simulink library "DatalogHandler"  (R2016b)
settings: Solver=VariableStepAuto  StartTime=0.0  StopTime=10.0  RelTol=1e-3
libraries: VariousLibrary x6, ConversionsLibrary x6, slrtlib x1
(part 2 of 2)

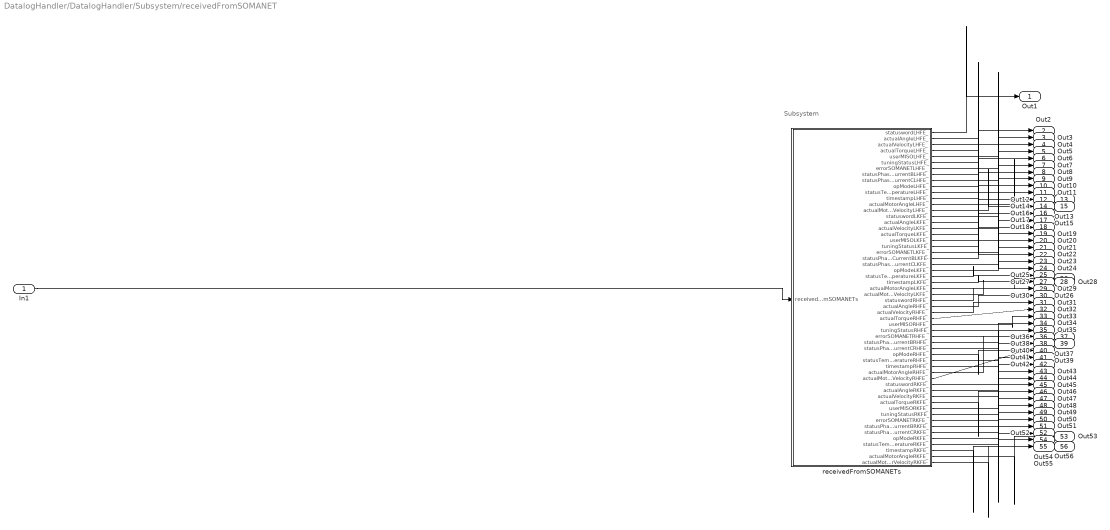
== system DatalogHandler/DatalogHandler/Subsystem/receivedFromSOMANET ==
  note: Subsystem
  In1 : Inport
  receivedFromSOMANETs : Subsystem
  Out1 : Outport
  Out2 : Outport  Port=2
  Out3 : Outport  Port=3
  Out4 : Outport  Port=4
  Out5 : Outport  Port=5
  Out6 : Outport  Port=6
  Out7 : Outport  Port=7
  Out8 : Outport  Port=8
  Out9 : Outport  Port=9
  Out10 : Outport  Port=10
  Out11 : Outport  Port=11
  Out12 : Outport  Port=12
  Out13 : Outport  Port=13
  Out14 : Outport  Port=14
  Out15 : Outport  Port=15
  Out16 : Outport  Port=16
  Out17 : Outport  Port=17
  Out18 : Outport  Port=18
  Out19 : Outport  Port=19
  Out20 : Outport  Port=20
  Out21 : Outport  Port=21
  Out22 : Outport  Port=22
  Out23 : Outport  Port=23
  Out24 : Outport  Port=24
  Out25 : Outport  Port=25
  Out26 : Outport  Port=26
  Out27 : Outport  Port=27
  Out28 : Outport  Port=28
  Out29 : Outport  Port=29
  Out30 : Outport  Port=30
  Out31 : Outport  Port=31
  Out32 : Outport  Port=32
  Out33 : Outport  Port=33
  Out34 : Outport  Port=34
  Out35 : Outport  Port=35
  Out36 : Outport  Port=36
  Out37 : Outport  Port=37
  Out38 : Outport  Port=38
  Out39 : Outport  Port=39
  Out40 : Outport  Port=40
  Out41 : Outport  Port=41
  Out42 : Outport  Port=42
  Out43 : Outport  Port=43
  Out44 : Outport  Port=44
  Out45 : Outport  Port=45
  Out46 : Outport  Port=46
  Out47 : Outport  Port=47
  Out48 : Outport  Port=48
  Out49 : Outport  Port=49
  Out50 : Outport  Port=50
  Out51 : Outport  Port=51
  Out52 : Outport  Port=52
  Out53 : Outport  Port=53
  Out54 : Outport  Port=54
  Out55 : Outport  Port=55
  Out56 : Outport  Port=56
  wires:
  receivedFromSOMANETs/34(tuningStatusRHFE_) -> Out34/1
  receivedFromSOMANETs/49(errorSOMANETRKFE_) -> Out49/1
  receivedFromSOMANETs/53(statusTemperatureRKFE_) -> Out54/1
  receivedFromSOMANETs/48(tuningStatusRKFE_) -> Out48/1
  receivedFromSOMANETs/38(opModeRHFE_) -> Out40/1
  receivedFromSOMANETs/51(statusPhaseCurrentCRKFE_) -> Out51/1
  receivedFromSOMANETs/39(statusTemperatureRHFE_) -> Out41/1
  receivedFromSOMANETs/47(userMISORKFE_) -> Out47/1
  receivedFromSOMANETs/45(actualVelocityRKFE_) -> Out45/1
  receivedFromSOMANETs/32(actualTorqueRHFE_) -> Out32/1
  receivedFromSOMANETs/46(actualTorqueRKFE_) -> Out46/1
  receivedFromSOMANETs/31(actualVelocityRHFE_) -> Out31/1
  receivedFromSOMANETs/44(actualAngleRKFE_) -> Out44/1
  receivedFromSOMANETs/43(statuswordRKFE_) -> Out43/1
  receivedFromSOMANETs/33(userMISORHFE_) -> Out33/1
  receivedFromSOMANETs/35(errorSOMANETRHFE_) -> Out35/1
  receivedFromSOMANETs/54(timestampRKFE_) -> Out55/1
  receivedFromSOMANETs/50(statusPhaseCurrentBRKFE_) -> Out50/1
  receivedFromSOMANETs/37(statusPhaseCurrentCRHFE_) -> Out38/1
  receivedFromSOMANETs/40(timestampRHFE_) -> Out42/1
  receivedFromSOMANETs/52(opModeRKFE_) -> Out52/1
  receivedFromSOMANETs/36(statusPhaseCurrentBRHFE_) -> Out36/1
  receivedFromSOMANETs/30(actualAngleRHFE_) -> Out30/1
  receivedFromSOMANETs/18(actualTorqueLKFE_) -> Out18/1
  receivedFromSOMANETs/1(statuswordLHFE_) -> Out1/1
  receivedFromSOMANETs/2(actualAngleLHFE_) -> Out2/1
  receivedFromSOMANETs/17(actualVelocityLKFE_) -> Out17/1
  receivedFromSOMANETs/11(statusTemperatureLHFE_) -> Out11/1
  receivedFromSOMANETs/10(opModeLHFE_) -> Out10/1
  receivedFromSOMANETs/21(errorSOMANETLKFE_) -> Out21/1
  receivedFromSOMANETs/15(statuswordLKFE_) -> Out14/1
  receivedFromSOMANETs/8(statusPhaseCurrentBLHFE_) -> Out8/1
  receivedFromSOMANETs/4(actualTorqueLHFE_) -> Out4/1
  receivedFromSOMANETs/12(timestampLHFE_) -> Out12/1
  receivedFromSOMANETs/5(userMISOLHFE_) -> Out5/1
  receivedFromSOMANETs/29(statuswordRHFE_) -> Out29/1
  receivedFromSOMANETs/24(opModeLKFE_) -> Out24/1
  receivedFromSOMANETs/3(actualVelocityLHFE_) -> Out3/1
  receivedFromSOMANETs/7(errorSOMANETLHFE_) -> Out7/1
  receivedFromSOMANETs/20(tuningStatusLKFE_) -> Out20/1
  receivedFromSOMANETs/9(statusPhaseCurrentCLHFE_) -> Out9/1
  receivedFromSOMANETs/26(timestampLKFE_) -> Out27/1
  receivedFromSOMANETs/6(tuningStatusLHFE_) -> Out6/1
  receivedFromSOMANETs/25(statusTemperatureLKFE_) -> Out25/1
  receivedFromSOMANETs/23(statusPhaseCurrentCLKFE_) -> Out23/1
  receivedFromSOMANETs/22(statusPhaseCurrentBLKFE-) -> Out22/1
  receivedFromSOMANETs/19(userMISOLKFE_) -> Out19/1
  receivedFromSOMANETs/16(actualAngleLKFE_) -> Out16/1
  receivedFromSOMANETs/13(actualMotorAngleLHFE_) -> Out13/1
  receivedFromSOMANETs/14(actualMotorVelocityLHFE_) -> Out15/1
  receivedFromSOMANETs/56(actualMotorVelocityRKFE-) -> Out56/1
  receivedFromSOMANETs/27(actualMotorAngleLKFE_) -> Out26/1
  receivedFromSOMANETs/55(actualMotorAngleRKFE_) -> Out53/1
  receivedFromSOMANETs/28(actualMotorVelocityLKFE_) -> Out28/1
  receivedFromSOMANETs/42(actualMotorVelocityRHFE_) -> Out39/1
  receivedFromSOMANETs/41(actualMotorAngleRHFE_) -> Out37/1
  In1/1 -> receivedFromSOMANETs/1(receivedFromSOMANETs)

== system DatalogHandler/DatalogHandler/Subsystem/sendToInputDevice ==
  In1 : Inport
  Bus Selector7 : BusSelector  OutputSignals=state,message
  messageToInputDevice : DataTypeConversion  OutDataTypeStr=double  RndMeth=Nearest
  stateToInputDevice : DataTypeConversion  OutDataTypeStr=double  RndMeth=Nearest
  Out1 : Outport
  Out2 : Outport  Port=2
  wires:
  messageToInputDevice/1 -> Out2/1
  stateToInputDevice/1 -> Out1/1
  In1/1 -> Bus Selector7/1
  Bus Selector7/1 -> stateToInputDevice/1  "<state>"
  Bus Selector7/2 -> messageToInputDevice/1  "<message>"

== system DatalogHandler/DatalogHandler/Subsystem/sendToPowerElectronics ==
  In1 : Inport
  Bus Selector9 : BusSelector  OutputSignals=sendToPDB.masterOP
  masterOP : DataTypeConversion  OutDataTypeStr=double  RndMeth=Nearest
  Out1 : Outport
  wires:
  masterOP/1 -> Out1/1
  In1/1 -> Bus Selector9/1
  Bus Selector9/1 -> masterOP/1  "<masterOP>"

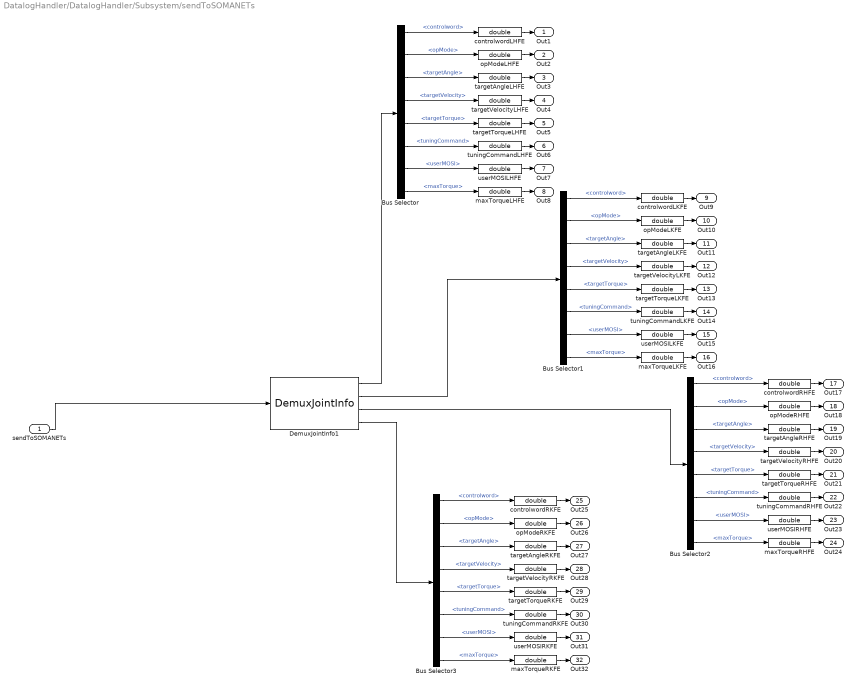
== system DatalogHandler/DatalogHandler/Subsystem/sendToSOMANETs ==
  sendToSOMANETs : Inport
  Bus Selector{,1..3} (4 alike) : BusSelector  OutputSignals=controlword,opMode,targetAngle,targetVelocity,targetTorque,tuningCommand,userMOSI,maxTorque
  DemuxJointInfo1 : VariousLibrary/DemuxJointInfo
  controlwordLHFE : DataTypeConversion  OutDataTypeStr=double  RndMeth=Nearest
  controlwordLKFE : DataTypeConversion  OutDataTypeStr=double  RndMeth=Nearest
  controlwordRHFE : DataTypeConversion  OutDataTypeStr=double  RndMeth=Nearest
  controlwordRKFE : DataTypeConversion  OutDataTypeStr=double  RndMeth=Nearest
  maxTorqueLHFE : DataTypeConversion  OutDataTypeStr=double  RndMeth=Nearest
  maxTorqueLKFE : DataTypeConversion  OutDataTypeStr=double  RndMeth=Nearest
  maxTorqueRHFE : DataTypeConversion  OutDataTypeStr=double  RndMeth=Nearest
  maxTorqueRKFE : DataTypeConversion  OutDataTypeStr=double  RndMeth=Nearest
  opModeLHFE : DataTypeConversion  OutDataTypeStr=double  RndMeth=Nearest
  opModeLKFE : DataTypeConversion  OutDataTypeStr=double  RndMeth=Nearest
  opModeRHFE : DataTypeConversion  OutDataTypeStr=double  RndMeth=Nearest
  opModeRKFE : DataTypeConversion  OutDataTypeStr=double  RndMeth=Nearest
  targetAngleLHFE : DataTypeConversion  OutDataTypeStr=double  RndMeth=Nearest
  targetAngleLKFE : DataTypeConversion  OutDataTypeStr=double  RndMeth=Nearest
  targetAngleRHFE : DataTypeConversion  OutDataTypeStr=double  RndMeth=Nearest
  targetAngleRKFE : DataTypeConversion  OutDataTypeStr=double  RndMeth=Nearest
  targetTorqueLHFE : DataTypeConversion  OutDataTypeStr=double  RndMeth=Nearest
  targetTorqueLKFE : DataTypeConversion  OutDataTypeStr=double  RndMeth=Nearest
  targetTorqueRHFE : DataTypeConversion  OutDataTypeStr=double  RndMeth=Nearest
  targetTorqueRKFE : DataTypeConversion  OutDataTypeStr=double  RndMeth=Nearest
  targetVelocityLHFE : DataTypeConversion  OutDataTypeStr=double  RndMeth=Nearest
  targetVelocityLKFE : DataTypeConversion  OutDataTypeStr=double  RndMeth=Nearest
  targetVelocityRHFE : DataTypeConversion  OutDataTypeStr=double  RndMeth=Nearest
  targetVelocityRKFE : DataTypeConversion  OutDataTypeStr=double  RndMeth=Nearest
  tuningCommandLHFE : DataTypeConversion  OutDataTypeStr=double  RndMeth=Nearest
  tuningCommandLKFE : DataTypeConversion  OutDataTypeStr=double  RndMeth=Nearest
  tuningCommandRHFE : DataTypeConversion  OutDataTypeStr=double  RndMeth=Nearest
  tuningCommandRKFE : DataTypeConversion  OutDataTypeStr=double  RndMeth=Nearest
  userMOSILHFE : DataTypeConversion  OutDataTypeStr=double  RndMeth=Nearest
  userMOSILKFE : DataTypeConversion  OutDataTypeStr=double  RndMeth=Nearest
  userMOSIRHFE : DataTypeConversion  OutDataTypeStr=double  RndMeth=Nearest
  userMOSIRKFE : DataTypeConversion  OutDataTypeStr=double  RndMeth=Nearest
  Out1 : Outport
  Out2 : Outport  Port=2
  Out3 : Outport  Port=3
  Out4 : Outport  Port=4
  Out5 : Outport  Port=5
  Out6 : Outport  Port=6
  Out7 : Outport  Port=7
  Out8 : Outport  Port=8
  Out9 : Outport  Port=9
  Out10 : Outport  Port=10
  Out11 : Outport  Port=11
  Out12 : Outport  Port=12
  Out13 : Outport  Port=13
  Out14 : Outport  Port=14
  Out15 : Outport  Port=15
  Out16 : Outport  Port=16
  Out17 : Outport  Port=17
  Out18 : Outport  Port=18
  Out19 : Outport  Port=19
  Out20 : Outport  Port=20
  Out21 : Outport  Port=21
  Out22 : Outport  Port=22
  Out23 : Outport  Port=23
  Out24 : Outport  Port=24
  Out25 : Outport  Port=25
  Out26 : Outport  Port=26
  Out27 : Outport  Port=27
  Out28 : Outport  Port=28
  Out29 : Outport  Port=29
  Out30 : Outport  Port=30
  Out31 : Outport  Port=31
  Out32 : Outport  Port=32
  wires:
  DemuxJointInfo1/4 -> Bus Selector3/1
  maxTorqueRKFE/1 -> Out32/1
  userMOSIRKFE/1 -> Out31/1
  tuningCommandRKFE/1 -> Out30/1
  targetTorqueRKFE/1 -> Out29/1
  targetVelocityRKFE/1 -> Out28/1
  targetAngleRKFE/1 -> Out27/1
  opModeRKFE/1 -> Out26/1
  controlwordRKFE/1 -> Out25/1
  Bus Selector3/8 -> maxTorqueRKFE/1  "<maxTorque>"
  Bus Selector3/7 -> userMOSIRKFE/1  "<userMOSI>"
  Bus Selector3/6 -> tuningCommandRKFE/1  "<tuningCommand>"
  Bus Selector3/5 -> targetTorqueRKFE/1  "<targetTorque>"
  Bus Selector3/4 -> targetVelocityRKFE/1  "<targetVelocity>"
  Bus Selector3/3 -> targetAngleRKFE/1  "<targetAngle>"
  Bus Selector3/2 -> opModeRKFE/1  "<opMode>"
  Bus Selector3/1 -> controlwordRKFE/1  "<controlword>"
  maxTorqueRHFE/1 -> Out24/1
  userMOSIRHFE/1 -> Out23/1
  tuningCommandRHFE/1 -> Out22/1
  targetTorqueRHFE/1 -> Out21/1
  targetVelocityRHFE/1 -> Out20/1
  targetAngleRHFE/1 -> Out19/1
  opModeRHFE/1 -> Out18/1
  controlwordRHFE/1 -> Out17/1
  Bus Selector2/8 -> maxTorqueRHFE/1  "<maxTorque>"
  Bus Selector2/7 -> userMOSIRHFE/1  "<userMOSI>"
  Bus Selector2/6 -> tuningCommandRHFE/1  "<tuningCommand>"
  Bus Selector2/5 -> targetTorqueRHFE/1  "<targetTorque>"
  Bus Selector2/4 -> targetVelocityRHFE/1  "<targetVelocity>"
  Bus Selector2/3 -> targetAngleRHFE/1  "<targetAngle>"
  Bus Selector2/2 -> opModeRHFE/1  "<opMode>"
  Bus Selector2/1 -> controlwordRHFE/1  "<controlword>"
  DemuxJointInfo1/3 -> Bus Selector2/1
  maxTorqueLKFE/1 -> Out16/1
  userMOSILKFE/1 -> Out15/1
  tuningCommandLKFE/1 -> Out14/1
  targetTorqueLKFE/1 -> Out13/1
  targetVelocityLKFE/1 -> Out12/1
  targetAngleLKFE/1 -> Out11/1
  opModeLKFE/1 -> Out10/1
  controlwordLKFE/1 -> Out9/1
  Bus Selector1/8 -> maxTorqueLKFE/1  "<maxTorque>"
  Bus Selector1/7 -> userMOSILKFE/1  "<userMOSI>"
  Bus Selector1/6 -> tuningCommandLKFE/1  "<tuningCommand>"
  Bus Selector1/5 -> targetTorqueLKFE/1  "<targetTorque>"
  Bus Selector1/4 -> targetVelocityLKFE/1  "<targetVelocity>"
  Bus Selector1/3 -> targetAngleLKFE/1  "<targetAngle>"
  Bus Selector1/2 -> opModeLKFE/1  "<opMode>"
  Bus Selector1/1 -> controlwordLKFE/1  "<controlword>"
  DemuxJointInfo1/2 -> Bus Selector1/1
  maxTorqueLHFE/1 -> Out8/1
  userMOSILHFE/1 -> Out7/1
  tuningCommandLHFE/1 -> Out6/1
  targetTorqueLHFE/1 -> Out5/1
  targetVelocityLHFE/1 -> Out4/1
  targetAngleLHFE/1 -> Out3/1
  opModeLHFE/1 -> Out2/1
  controlwordLHFE/1 -> Out1/1
  Bus Selector/8 -> maxTorqueLHFE/1  "<maxTorque>"
  Bus Selector/7 -> userMOSILHFE/1  "<userMOSI>"
  Bus Selector/6 -> tuningCommandLHFE/1  "<tuningCommand>"
  Bus Selector/5 -> targetTorqueLHFE/1  "<targetTorque>"
  Bus Selector/4 -> targetVelocityLHFE/1  "<targetVelocity>"
  Bus Selector/3 -> targetAngleLHFE/1  "<targetAngle>"
  Bus Selector/2 -> opModeLHFE/1  "<opMode>"
  Bus Selector/1 -> controlwordLHFE/1  "<controlword>"
  sendToSOMANETs/1 -> DemuxJointInfo1/1
  DemuxJointInfo1/1 -> Bus Selector/1

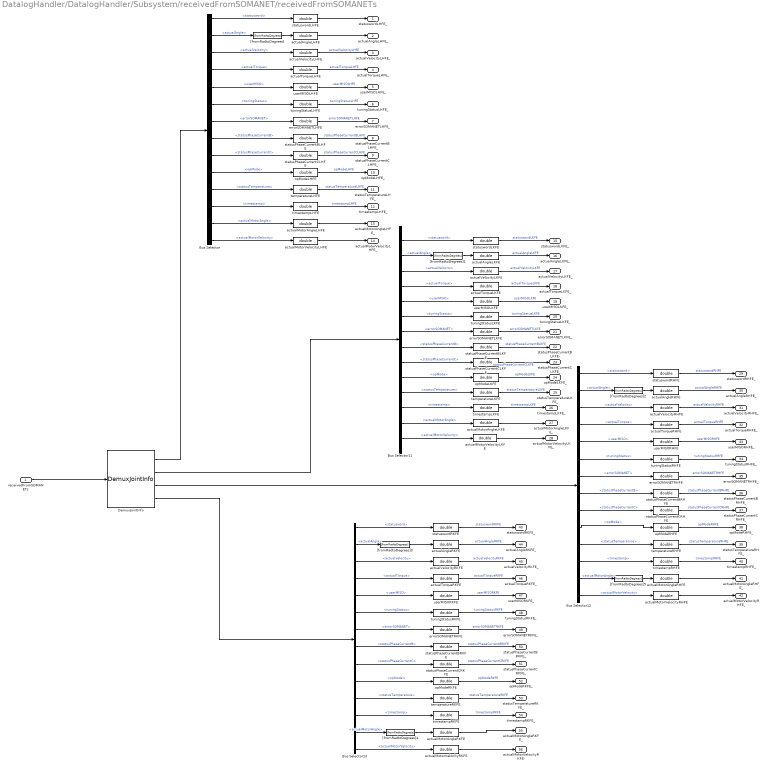
== system DatalogHandler/DatalogHandler/Subsystem/receivedFromSOMANET/receivedFromSOMANETs ==
  receivedFromSOMANETs : Inport
  Bus Selector{,11..13} (4 alike) : BusSelector  OutputSignals=statusword,actualAngle,actualVelocity,actualTorque,userMISO,tuningStatus,errorSOMANET,statusPhaseCurrentB,statusPhaseCurrentC,opMode,statusTemperature,timestamp,actualMotorAngle,actualMotorVelocity
  DemuxJointInfo : VariousLibrary/DemuxJointInfo
  [fromRadtoDegrees]{,1..5} (6 alike) : ConversionsLibrary/[fromRadtoDegrees]
  actualAngleLHFE : DataTypeConversion  OutDataTypeStr=double  RndMeth=Nearest
  actualAngleLKFE : DataTypeConversion  OutDataTypeStr=double  RndMeth=Nearest
  actualAngleRHFE : DataTypeConversion  OutDataTypeStr=double  RndMeth=Nearest
  actualAngleRKFE : DataTypeConversion  OutDataTypeStr=double  RndMeth=Nearest
  actualMotorAngleLHFE : DataTypeConversion  OutDataTypeStr=double  RndMeth=Nearest
  actualMotorAngleLKFE : DataTypeConversion  OutDataTypeStr=double  RndMeth=Nearest
  actualMotorAngleRHFE : DataTypeConversion  OutDataTypeStr=double  RndMeth=Nearest
  actualMotorAngleRKFE : DataTypeConversion  OutDataTypeStr=double  RndMeth=Nearest
  actualMotorVelocityLHFE : DataTypeConversion  OutDataTypeStr=double  RndMeth=Nearest
  actualMotorVelocityLKFE : DataTypeConversion  OutDataTypeStr=double  RndMeth=Nearest
  actualMotorVelocityRHFE : DataTypeConversion  OutDataTypeStr=double  RndMeth=Nearest
  actualMotorVelocityRKFE : DataTypeConversion  OutDataTypeStr=double  RndMeth=Nearest
  actualTorqueLHFE : DataTypeConversion  OutDataTypeStr=double  RndMeth=Nearest
  actualTorqueLKFE : DataTypeConversion  OutDataTypeStr=double  RndMeth=Nearest
  actualTorqueRHFE : DataTypeConversion  OutDataTypeStr=double  RndMeth=Nearest
  actualTorqueRKFE : DataTypeConversion  OutDataTypeStr=double  RndMeth=Nearest
  actualVelocityLHFE : DataTypeConversion  OutDataTypeStr=double  RndMeth=Nearest
  actualVelocityLKFE : DataTypeConversion  OutDataTypeStr=double  RndMeth=Nearest
  actualVelocityRHFE : DataTypeConversion  OutDataTypeStr=double  RndMeth=Nearest
  actualVelocityRKFE : DataTypeConversion  OutDataTypeStr=double  RndMeth=Nearest
  errorSOMANETLHFE : DataTypeConversion  OutDataTypeStr=double  RndMeth=Nearest
  errorSOMANETLKFE : DataTypeConversion  OutDataTypeStr=double  RndMeth=Nearest
  errorSOMANETRHFE : DataTypeConversion  OutDataTypeStr=double  RndMeth=Nearest
  errorSOMANETRKFE : DataTypeConversion  OutDataTypeStr=double  RndMeth=Nearest
  opModeLHFE : DataTypeConversion  OutDataTypeStr=double  RndMeth=Nearest
  opModeLKFE : DataTypeConversion  OutDataTypeStr=double  RndMeth=Nearest
  opModeRHFE : DataTypeConversion  OutDataTypeStr=double  RndMeth=Nearest
  opModeRKFE : DataTypeConversion  OutDataTypeStr=double  RndMeth=Nearest
  statusPhaseCurrentBLHFE : DataTypeConversion  OutDataTypeStr=double  RndMeth=Nearest
  statusPhaseCurrentBLKFE : DataTypeConversion  OutDataTypeStr=double  RndMeth=Nearest
  statusPhaseCurrentBRHFE : DataTypeConversion  OutDataTypeStr=double  RndMeth=Nearest
  statusPhaseCurrentBRKFE : DataTypeConversion  OutDataTypeStr=double  RndMeth=Nearest
  statusPhaseCurrentCLHFE : DataTypeConversion  OutDataTypeStr=double  RndMeth=Nearest
  statusPhaseCurrentCLKFE : DataTypeConversion  OutDataTypeStr=double  RndMeth=Nearest
  statusPhaseCurrentCRHFE : DataTypeConversion  OutDataTypeStr=double  RndMeth=Nearest
  statusPhaseCurrentCRKFE : DataTypeConversion  OutDataTypeStr=double  RndMeth=Nearest
  statuswordLHFE : DataTypeConversion  OutDataTypeStr=double  RndMeth=Nearest
  statuswordLKFE : DataTypeConversion  OutDataTypeStr=double  RndMeth=Nearest
  statuswordRHFE : DataTypeConversion  OutDataTypeStr=double  RndMeth=Nearest
  statuswordRKFE : DataTypeConversion  OutDataTypeStr=double  RndMeth=Nearest
  temperatureLHFE : DataTypeConversion  OutDataTypeStr=double  RndMeth=Nearest
  temperatureLKFE : DataTypeConversion  OutDataTypeStr=double  RndMeth=Nearest
  temperatureRHFE : DataTypeConversion  OutDataTypeStr=double  RndMeth=Nearest
  temperatureRKFE : DataTypeConversion  OutDataTypeStr=double  RndMeth=Nearest
  timestampLHFE : DataTypeConversion  OutDataTypeStr=double  RndMeth=Nearest
  timestampLKFE : DataTypeConversion  OutDataTypeStr=double  RndMeth=Nearest
  timestampRHFE : DataTypeConversion  OutDataTypeStr=double  RndMeth=Nearest
  timestampRKFE : DataTypeConversion  OutDataTypeStr=double  RndMeth=Nearest
  tuningStatusLHFE : DataTypeConversion  OutDataTypeStr=double  RndMeth=Nearest
  tuningStatusLKFE : DataTypeConversion  OutDataTypeStr=double  RndMeth=Nearest
  tuningStatusRHFE : DataTypeConversion  OutDataTypeStr=double  RndMeth=Nearest
  tuningStatusRKFE : DataTypeConversion  OutDataTypeStr=double  RndMeth=Nearest
  userMISOLHFE : DataTypeConversion  OutDataTypeStr=double  RndMeth=Nearest
  userMISOLKFE : DataTypeConversion  OutDataTypeStr=double  RndMeth=Nearest
  userMISORHFE : DataTypeConversion  OutDataTypeStr=double  RndMeth=Nearest
  userMISORKFE : DataTypeConversion  OutDataTypeStr=double  RndMeth=Nearest
  statuswordLHFE_ : Outport
  actualAngleLHFE_ : Outport  Port=2
  actualVelocityLHFE_ : Outport  Port=3
  actualTorqueLHFE_ : Outport  Port=4
  userMISOLHFE_ : Outport  Port=5
  tuningStatusLHFE_ : Outport  Port=6
  errorSOMANETLHFE_ : Outport  Port=7
  statusPhaseCurrentBLHFE_ : Outport  Port=8
  statusPhaseCurrentCLHFE_ : Outport  Port=9
  opModeLHFE_ : Outport  Port=10
  statusTemperatureLHFE_ : Outport  Port=11
  timestampLHFE_ : Outport  Port=12
  actualMotorAngleLHFE_ : Outport  Port=13
  actualMotorVelocityLHFE_ : Outport  Port=14
  statuswordLKFE_ : Outport  Port=15
  actualAngleLKFE_ : Outport  Port=16
  actualVelocityLKFE_ : Outport  Port=17
  actualTorqueLKFE_ : Outport  Port=18
  userMISOLKFE_ : Outport  Port=19
  tuningStatusLKFE_ : Outport  Port=20
  errorSOMANETLKFE_ : Outport  Port=21
  statusPhaseCurrentBLKFE- : Outport  Port=22
  statusPhaseCurrentCLKFE_ : Outport  Port=23
  opModeLKFE_ : Outport  Port=24
  statusTemperatureLKFE_ : Outport  Port=25
  timestampLKFE_ : Outport  Port=26
  actualMotorAngleLKFE_ : Outport  Port=27
  actualMotorVelocityLKFE_ : Outport  Port=28
  statuswordRHFE_ : Outport  Port=29
  actualAngleRHFE_ : Outport  Port=30
  actualVelocityRHFE_ : Outport  Port=31
  actualTorqueRHFE_ : Outport  Port=32
  userMISORHFE_ : Outport  Port=33
  tuningStatusRHFE_ : Outport  Port=34
  errorSOMANETRHFE_ : Outport  Port=35
  statusPhaseCurrentBRHFE_ : Outport  Port=36
  statusPhaseCurrentCRHFE_ : Outport  Port=37
  opModeRHFE_ : Outport  Port=38
  statusTemperatureRHFE_ : Outport  Port=39
  timestampRHFE_ : Outport  Port=40
  actualMotorAngleRHFE_ : Outport  Port=41
  actualMotorVelocityRHFE_ : Outport  Port=42
  statuswordRKFE_ : Outport  Port=43
  actualAngleRKFE_ : Outport  Port=44
  actualVelocityRKFE_ : Outport  Port=45
  actualTorqueRKFE_ : Outport  Port=46
  userMISORKFE_ : Outport  Port=47
  tuningStatusRKFE_ : Outport  Port=48
  errorSOMANETRKFE_ : Outport  Port=49
  statusPhaseCurrentBRKFE_ : Outport  Port=50
  statusPhaseCurrentCRKFE_ : Outport  Port=51
  opModeRKFE_ : Outport  Port=52
  statusTemperatureRKFE_ : Outport  Port=53
  timestampRKFE_ : Outport  Port=54
  actualMotorAngleRKFE_ : Outport  Port=55
  actualMotorVelocityRKFE- : Outport  Port=56
  wires:
  "[fromRadtoDegrees]5"/1 -> actualMotorAngleRHFE/1
  "[fromRadtoDegrees]4"/1 -> actualMotorAngleRKFE/1
  actualMotorVelocityRKFE/1 -> actualMotorVelocityRKFE-/1
  actualMotorAngleRKFE/1 -> actualMotorAngleRKFE_/1
  Bus Selector13/14 -> actualMotorVelocityRKFE/1  "<actualMotorVelocity>"
  Bus Selector13/13 -> "[fromRadtoDegrees]4"/1  "<actualMotorAngle>"
  actualMotorAngleRHFE/1 -> actualMotorAngleRHFE_/1
  actualMotorVelocityRHFE/1 -> actualMotorVelocityRHFE_/1
  Bus Selector12/14 -> actualMotorVelocityRHFE/1  "<actualMotorVelocity>"
  Bus Selector12/13 -> "[fromRadtoDegrees]5"/1  "<actualMotorAngle>"
  actualMotorVelocityLKFE/1 -> actualMotorVelocityLKFE_/1
  actualMotorAngleLKFE/1 -> actualMotorAngleLKFE_/1
  Bus Selector11/14 -> actualMotorVelocityLKFE/1  "<actualMotorVelocity>"
  Bus Selector11/13 -> actualMotorAngleLKFE/1  "<actualMotorAngle>"
  actualMotorVelocityLHFE/1 -> actualMotorVelocityLHFE_/1
  actualMotorAngleLHFE/1 -> actualMotorAngleLHFE_/1
  Bus Selector/13 -> actualMotorAngleLHFE/1  "<actualMotorAngle>"
  Bus Selector/14 -> actualMotorVelocityLHFE/1  "<actualMotorVelocity>"
  Bus Selector/2 -> "[fromRadtoDegrees]"/1  "<actualAngle>"
  Bus Selector/6 -> tuningStatusLHFE/1  "<tuningStatus>"
  Bus Selector/3 -> actualVelocityLHFE/1  "<actualVelocity>"
  "[fromRadtoDegrees]"/1 -> actualAngleLHFE/1
  "[fromRadtoDegrees]3"/1 -> actualAngleRKFE/1
  "[fromRadtoDegrees]2"/1 -> actualAngleRHFE/1
  statusPhaseCurrentCLHFE/1 -> statusPhaseCurrentCLHFE_/1  "statusPhaseCurrentCLHFE"
  statusPhaseCurrentBLHFE/1 -> statusPhaseCurrentBLHFE_/1  "statusPhaseCurrentBLHFE"
  DemuxJointInfo/2 -> Bus Selector11/1
  DemuxJointInfo/4 -> Bus Selector13/1
  tuningStatusLHFE/1 -> tuningStatusLHFE_/1  "tuningStatusLHFE"
  statuswordLHFE/1 -> statuswordLHFE_/1
  actualAngleLHFE/1 -> actualAngleLHFE_/1
  actualTorqueLHFE/1 -> actualTorqueLHFE_/1  "actualTorqueLHFE"
  errorSOMANETLHFE/1 -> errorSOMANETLHFE_/1  "errorSOMANETLHFE"
  actualTorqueRHFE/1 -> actualTorqueRHFE_/1  "actualTorqueRHFE"
  statusPhaseCurrentCRHFE/1 -> statusPhaseCurrentCRHFE_/1  "statusPhaseCurrentCRHFE"
  Bus Selector12/7 -> errorSOMANETRHFE/1  "<errorSOMANET>"
  Bus Selector12/4 -> actualTorqueRHFE/1  "<actualTorque>"
  opModeRHFE/1 -> opModeRHFE_/1  "opModeRHFE"
  opModeLHFE/1 -> opModeLHFE_/1  "opModeLHFE"
  userMISORHFE/1 -> userMISORHFE_/1  "userMISORHFE"
  statuswordRHFE/1 -> statuswordRHFE_/1  "statuswordRHFE"
  Bus Selector12/8 -> statusPhaseCurrentBRHFE/1  "<statusPhaseCurrentB>"
  actualVelocityRHFE/1 -> actualVelocityRHFE_/1  "actualVelocityRHFE"
  timestampRHFE/1 -> timestampRHFE_/1  "timestampRHFE"
  Bus Selector12/9 -> statusPhaseCurrentCRHFE/1  "<statusPhaseCurrentC>"
  temperatureRHFE/1 -> statusTemperatureRHFE_/1  "statusTemperatureRHFE"
  statusPhaseCurrentBRHFE/1 -> statusPhaseCurrentBRHFE_/1  "statusPhaseCurrentBRHFE"
  errorSOMANETRHFE/1 -> errorSOMANETRHFE_/1  "errorSOMANETRHFE"
  tuningStatusRHFE/1 -> tuningStatusRHFE_/1  "tuningStatusRHFE"
  actualAngleRHFE/1 -> actualAngleRHFE_/1  "actualAngleRHFE"
  Bus Selector12/10 -> opModeRHFE/1  "<opMode>"
  Bus Selector12/3 -> actualVelocityRHFE/1  "<actualVelocity>"
  Bus Selector12/2 -> "[fromRadtoDegrees]2"/1  "<actualAngle>"
  Bus Selector12/12 -> timestampRHFE/1  "<timestamp>"
  Bus Selector12/11 -> temperatureRHFE/1  "<statusTemperature>"
  Bus Selector12/6 -> tuningStatusRHFE/1  "<tuningStatus>"
  Bus Selector12/5 -> userMISORHFE/1  "<userMISO>"
  Bus Selector12/1 -> statuswordRHFE/1  "<statusword>"
  temperatureLHFE/1 -> statusTemperatureLHFE_/1  "statusTemperatureLHFE"
  timestampLHFE/1 -> timestampLHFE_/1  "timestampLHFE"
  actualVelocityLHFE/1 -> actualVelocityLHFE_/1  "actualVelocityLHFE"
  Bus Selector11/4 -> actualTorqueLKFE/1  "<actualTorque>"
  Bus Selector11/12 -> timestampLKFE/1  "<timestamp>"
  Bus Selector11/3 -> actualVelocityLKFE/1  "<actualVelocity>"
  Bus Selector11/11 -> temperatureLKFE/1  "<statusTemperature>"
  opModeLKFE/1 -> opModeLKFE_/1  "opModeLKFE"
  statuswordLKFE/1 -> statuswordLKFE_/1  "statuswordLKFE"
  Bus Selector11/8 -> statusPhaseCurrentBLKFE/1  "<statusPhaseCurrentB>"
  Bus Selector11/6 -> tuningStatusLKFE/1  "<tuningStatus>"
  statusPhaseCurrentBLKFE/1 -> statusPhaseCurrentBLKFE-/1  "statusPhaseCurrentBLKFE"
  actualAngleLKFE/1 -> actualAngleLKFE_/1  "actualAngleLKFE"
  Bus Selector11/2 -> "[fromRadtoDegrees]1"/1  "<actualAngle>"
  Bus Selector11/5 -> userMISOLKFE/1  "<userMISO>"
  Bus Selector11/7 -> errorSOMANETLKFE/1  "<errorSOMANET>"
  tuningStatusLKFE/1 -> tuningStatusLKFE_/1  "tuningStatusLKFE"
  timestampLKFE/1 -> timestampLKFE_/1  "timestampLKFE"
  temperatureLKFE/1 -> statusTemperatureLKFE_/1  "statusTemperatureLKFE"
  statusPhaseCurrentCLKFE/1 -> statusPhaseCurrentCLKFE_/1  "statusPhaseCurrentCLKFE"
  errorSOMANETLKFE/1 -> errorSOMANETLKFE_/1  "errorSOMANETLKFE"
  userMISOLKFE/1 -> userMISOLKFE_/1  "userMISOLKFE"
  actualTorqueLKFE/1 -> actualTorqueLKFE_/1  "actualTorqueLKFE"
  userMISOLHFE/1 -> userMISOLHFE_/1  "userMISOLHFE"
  actualVelocityLKFE/1 -> actualVelocityLKFE_/1  "actualVelocityLKFE"
  Bus Selector11/10 -> opModeLKFE/1  "<opMode>"
  Bus Selector11/9 -> statusPhaseCurrentCLKFE/1  "<statusPhaseCurrentC>"
  Bus Selector11/1 -> statuswordLKFE/1  "<statusword>"
  Bus Selector/5 -> userMISOLHFE/1  "<userMISO>"
  DemuxJointInfo/3 -> Bus Selector12/1
  "[fromRadtoDegrees]1"/1 -> actualAngleLKFE/1
  Bus Selector/1 -> statuswordLHFE/1  "<statusword>"
  Bus Selector/10 -> opModeLHFE/1  "<opMode>"
  Bus Selector/9 -> statusPhaseCurrentCLHFE/1  "<statusPhaseCurrentC>"
  actualTorqueRKFE/1 -> actualTorqueRKFE_/1  "actualTorqueRKFE"
  timestampRKFE/1 -> timestampRKFE_/1  "timestampRKFE"
  statusPhaseCurrentBRKFE/1 -> statusPhaseCurrentBRKFE_/1  "statusPhaseCurrentBRKFE"
  actualVelocityRKFE/1 -> actualVelocityRKFE_/1  "actualVelocityRKFE"
  Bus Selector13/10 -> opModeRKFE/1  "<opMode>"
  actualAngleRKFE/1 -> actualAngleRKFE_/1  "actualAngleRKFE"
  errorSOMANETRKFE/1 -> errorSOMANETRKFE_/1  "errorSOMANETRKFE"
  statusPhaseCurrentCRKFE/1 -> statusPhaseCurrentCRKFE_/1  "statusPhaseCurrentCRKFE"
  Bus Selector13/12 -> timestampRKFE/1  "<timestamp>"
  userMISORKFE/1 -> userMISORKFE_/1  "userMISORKFE"
  tuningStatusRKFE/1 -> tuningStatusRKFE_/1  "tuningStatusRKFE"
  temperatureRKFE/1 -> statusTemperatureRKFE_/1  "statusTemperatureRKFE"
  statuswordRKFE/1 -> statuswordRKFE_/1  "statuswordRKFE"
  Bus Selector13/11 -> temperatureRKFE/1  "<statusTemperature>"
  opModeRKFE/1 -> opModeRKFE_/1  "opModeRKFE"
  Bus Selector13/8 -> statusPhaseCurrentBRKFE/1  "<statusPhaseCurrentB>"
  Bus Selector13/9 -> statusPhaseCurrentCRKFE/1  "<statusPhaseCurrentC>"
  Bus Selector13/3 -> actualVelocityRKFE/1  "<actualVelocity>"
  Bus Selector/8 -> statusPhaseCurrentBLHFE/1  "<statusPhaseCurrentB>"
  Bus Selector13/4 -> actualTorqueRKFE/1  "<actualTorque>"
  Bus Selector13/7 -> errorSOMANETRKFE/1  "<errorSOMANET>"
  Bus Selector13/6 -> tuningStatusRKFE/1  "<tuningStatus>"
  Bus Selector13/5 -> userMISORKFE/1  "<userMISO>"
  Bus Selector13/1 -> statuswordRKFE/1  "<statusword>"
  Bus Selector/7 -> errorSOMANETLHFE/1  "<errorSOMANET>"
  Bus Selector13/2 -> "[fromRadtoDegrees]3"/1  "<actualAngle>"
  Bus Selector/4 -> actualTorqueLHFE/1  "<actualTorque>"
  Bus Selector/12 -> timestampLHFE/1  "<timestamp>"
  Bus Selector/11 -> temperatureLHFE/1  "<statusTemperature>"
  DemuxJointInfo/1 -> Bus Selector/1
  receivedFromSOMANETs/1 -> DemuxJointInfo/1

== matlab function DatalogHandler/Subsystem/miscDataSOMANET/MATLAB Function ==
  data: maxI2tSurface input; maxI2tSurfaceLHFE output; maxI2tSurfaceLKFE output; maxI2tSurfaceRHFE output; maxI2tSurfaceRKFE output
function [maxI2tSurfaceLHFE,maxI2tSurfaceLKFE,maxI2tSurfaceRHFE,maxI2tSurfaceRKFE]= fcn(maxI2tSurface)
maxI2tSurfaceLHFE = maxI2tSurface;
maxI2tSurfaceLKFE = maxI2tSurface;
maxI2tSurfaceRHFE = maxI2tSurface;
maxI2tSurfaceRKFE = maxI2tSurface;
